simulink library "ShutdownHandler"  (R2016b)
settings: Solver=VariableStepAuto  StartTime=0.0  StopTime=10.0  RelTol=1e-3
undefined symbols (not defined in the file or in its folder): ExoskeletonState
libraries: simulink x1
settings Model: Creator=march  LastModifiedBy=march

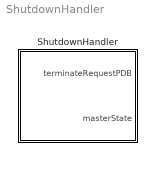
== system ShutdownHandler ==
  ShutdownHandler : Subsystem

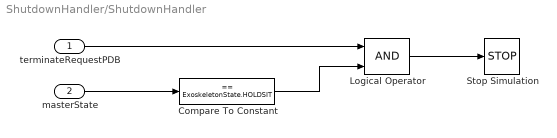
== system ShutdownHandler/ShutdownHandler ==
  terminateRequestPDB : Inport
  masterState : Inport  Port=2
  Compare To Constant : simulink/Logic and Bit Operations/Compare To Constant  relop===  const=ExoskeletonState.HOLDSIT  OutDataTypeStr=boolean
  Logical Operator : Logic  AllPortsSameDT=off  OutDataTypeStr=boolean
  Stop Simulation : Stop
  wires:
  masterState/1 -> Compare To Constant/1
  terminateRequestPDB/1 -> Logical Operator/1
  Compare To Constant/1 -> Logical Operator/2
  Logical Operator/1 -> Stop Simulation/1
